simulink model "CM745A_Sci30CfgAndUse"  (R2013b)
settings: Solver=ode45  StartTime=0.0  StopTime=10.0  RelTol=1e-3
libraries: simulink x12
(part 2 of 3)

== system CM745A_Sci30CfgAndUse/Sci30CfgAndUse/Sci30CfgAndUsePer1/Update DTS registers/If Action Subsystem3 ==
  Action Port : ActionPort  ActionType=then
  Add1 : Sum  OutDataTypeStr=Inherit: Inherit via back propagation
  Constant : Constant  Value=0
  Constant1 : Constant  Value=0
  Constant4 : Constant  OutDataTypeStr=uint8
  CopyRight2 : Subsystem  Description=|  mask(Copyright Information){none=on}
      | Copyright info block.                                               
      |                                                                     
      | Place copyright information at the top of every subsystem in design.
      mask prompts: none "No parameters"
      mask help: Place copyright information at the top of every subsystem in design.
      mask Display:
      | NxtrConf = 'Nexteer Confidential';
      | 
      | sys = bdroot; %handle for the current model ("system")
      | first = get_param(sys,'Created');
      | first = first(end-3:end);  %year is last four digits
      | 
      | last = get_param(sys,'LastModifiedDate');
      | if isempty(last)
      |     last = datestr(now,'yyyy');
      | else
      |     last = last(end-3:end);
      | end
      | 
      | if strcmp(first,last)
      |     fprintf('%s -- Copyright %s Nexteer',NxtrConf,first)
      | else
      |     fprintf('%s -- %s%s- %s Nexteer',NxtrConf,char(169),first,last)
      | end
  Data Store Read5 : DataStoreRead  DataStoreName=SciDiagcOvrrunErrCntr
  Data Store Write3 : DataStoreWrite  DataStoreName=SciDiagcOvrrunErrCntr
  RegOutpSCI30ORER : Terminator
  RegOutpSCI30RDRF : Terminator
  wires:
  Constant/1 -> RegOutpSCI30ORER/1
  Constant1/1 -> RegOutpSCI30RDRF/1
  Data Store Read5/1 -> Add1/1
  Add1/1 -> Data Store Write3/1
  Constant4/1 -> Add1/2

== system CM745A_Sci30CfgAndUse/Sci30CfgAndUse/Sci30CfgAndUsePer1/Update DTS registers/If Action Subsystem4 ==
  Action Port : ActionPort  ActionType=then
  Add1 : Sum  OutDataTypeStr=Inherit: Inherit via back propagation
  Constant : Constant  Value=0
  Constant4 : Constant  OutDataTypeStr=uint8
  CopyRight2 : Subsystem  Description=|  mask(Copyright Information){none=on}
      | Copyright info block.                                               
      |                                                                     
      | Place copyright information at the top of every subsystem in design.
      mask prompts: none "No parameters"
      mask help: Place copyright information at the top of every subsystem in design.
      mask Display:
      | NxtrConf = 'Nexteer Confidential';
      | 
      | sys = bdroot; %handle for the current model ("system")
      | first = get_param(sys,'Created');
      | first = first(end-3:end);  %year is last four digits
      | 
      | last = get_param(sys,'LastModifiedDate');
      | if isempty(last)
      |     last = datestr(now,'yyyy');
      | else
      |     last = last(end-3:end);
      | end
      | 
      | if strcmp(first,last)
      |     fprintf('%s -- Copyright %s Nexteer',NxtrConf,first)
      | else
      |     fprintf('%s -- %s%s- %s Nexteer',NxtrConf,char(169),first,last)
      | end
  Data Store Read5 : DataStoreRead  DataStoreName=SciDiagcParErrCntr
  Data Store Write3 : DataStoreWrite  DataStoreName=SciDiagcParErrCntr
  RegOutpSCI30PER : Terminator
  wires:
  Constant/1 -> RegOutpSCI30PER/1
  Data Store Read5/1 -> Add1/1
  Add1/1 -> Data Store Write3/1
  Constant4/1 -> Add1/2

== system CM745A_Sci30CfgAndUse/Sci30CfgAndUse/Sci30CfgAndUsePer1/Update DTS registers/If Action Subsystem5 ==
  Action Port : ActionPort  ActionType=then
  Add1 : Sum  OutDataTypeStr=Inherit: Inherit via back propagation
  Constant : Constant  Value=0
  Constant4 : Constant  OutDataTypeStr=uint8
  CopyRight2 : Subsystem  Description=|  mask(Copyright Information){none=on}
      | Copyright info block.                                               
      |                                                                     
      | Place copyright information at the top of every subsystem in design.
      mask prompts: none "No parameters"
      mask help: Place copyright information at the top of every subsystem in design.
      mask Display:
      | NxtrConf = 'Nexteer Confidential';
      | 
      | sys = bdroot; %handle for the current model ("system")
      | first = get_param(sys,'Created');
      | first = first(end-3:end);  %year is last four digits
      | 
      | last = get_param(sys,'LastModifiedDate');
      | if isempty(last)
      |     last = datestr(now,'yyyy');
      | else
      |     last = last(end-3:end);
      | end
      | 
      | if strcmp(first,last)
      |     fprintf('%s -- Copyright %s Nexteer',NxtrConf,first)
      | else
      |     fprintf('%s -- %s%s- %s Nexteer',NxtrConf,char(169),first,last)
      | end
  Data Store Read5 : DataStoreRead  DataStoreName=SciDiagcFrmErrCntr
  Data Store Write3 : DataStoreWrite  DataStoreName=SciDiagcFrmErrCntr
  RegOutpSCI30FER : Terminator
  wires:
  Constant/1 -> RegOutpSCI30FER/1
  Data Store Read5/1 -> Add1/1
  Add1/1 -> Data Store Write3/1
  Constant4/1 -> Add1/2

== system CM745A_Sci30CfgAndUse/Sci30CfgAndUse/Sci30CfgAndUsePer2/GetTxRateGroup/CopyRight2 ==

== system CM745A_Sci30CfgAndUse/Sci30CfgAndUse/Sci30CfgAndUsePer2/Sci30Transmit/CopyRight2 ==

== system CM745A_Sci30CfgAndUse/Sci30CfgAndUse/Sci30CfgAndUsePer2/Sci30Transmit/If Action Subsystem ==
  Action Port : ActionPort  ActionType=then
  Constant : Constant  Value=0  OutDataTypeStr=boolean
  Constant1 : Constant  Value=0  OutDataTypeStr=uint8
  CopyRight2 : Subsystem  Description=|  mask(Copyright Information){none=on}
      | Copyright info block.                                               
      |                                                                     
      | Place copyright information at the top of every subsystem in design.
      mask prompts: none "No parameters"
      mask help: Place copyright information at the top of every subsystem in design.
      mask Display:
      | NxtrConf = 'Nexteer Confidential';
      | 
      | sys = bdroot; %handle for the current model ("system")
      | first = get_param(sys,'Created');
      | first = first(end-3:end);  %year is last four digits
      | 
      | last = get_param(sys,'LastModifiedDate');
      | if isempty(last)
      |     last = datestr(now,'yyyy');
      | else
      |     last = last(end-3:end);
      | end
      | 
      | if strcmp(first,last)
      |     fprintf('%s -- Copyright %s Nexteer',NxtrConf,first)
      | else
      |     fprintf('%s -- %s%s- %s Nexteer',NxtrConf,char(169),first,last)
      | end
  Data Store Write : DataStoreWrite  DataStoreName=SciTxSigGroupCnt
  Data Store Write1 : DataStoreWrite  DataStoreName=SciGlbTxCnt
  IMCARBN_NROF2MILLISECRATEGROUP_CNT_U08 : Constant  Value=0  OutDataTypeStr=uint8
  While Iterator Subsystem : Subsystem  TreatAsAtomicUnit=on
  wires:
  Constant/1 -> While Iterator Subsystem/1(IC)
  Constant1/1 -> Data Store Write/1
  IMCARBN_NROF2MILLISECRATEGROUP_CNT_U08/1 -> Data Store Write1/1

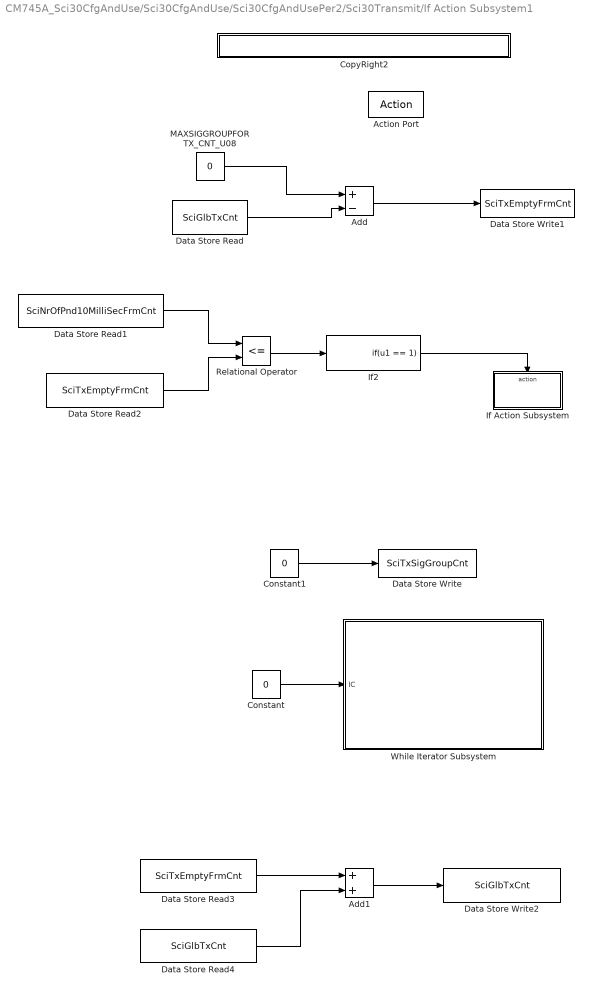
== system CM745A_Sci30CfgAndUse/Sci30CfgAndUse/Sci30CfgAndUsePer2/Sci30Transmit/If Action Subsystem1 ==
  Action Port : ActionPort  ActionType=then
  Add : Sum  Inputs=+-
  Add1 : Sum
  Constant : Constant  Value=0  OutDataTypeStr=boolean
  Constant1 : Constant  Value=0  OutDataTypeStr=uint8
  CopyRight2 : Subsystem  Description=|  mask(Copyright Information){none=on}
      | Copyright info block.                                               
      |                                                                     
      | Place copyright information at the top of every subsystem in design.
      mask prompts: none "No parameters"
      mask help: Place copyright information at the top of every subsystem in design.
      mask Display:
      | NxtrConf = 'Nexteer Confidential';
      | 
      | sys = bdroot; %handle for the current model ("system")
      | first = get_param(sys,'Created');
      | first = first(end-3:end);  %year is last four digits
      | 
      | last = get_param(sys,'LastModifiedDate');
      | if isempty(last)
      |     last = datestr(now,'yyyy');
      | else
      |     last = last(end-3:end);
      | end
      | 
      | if strcmp(first,last)
      |     fprintf('%s -- Copyright %s Nexteer',NxtrConf,first)
      | else
      |     fprintf('%s -- %s%s- %s Nexteer',NxtrConf,char(169),first,last)
      | end
  Data Store Read : DataStoreRead  DataStoreName=SciGlbTxCnt
  Data Store Read1 : DataStoreRead  DataStoreName=SciNrOfPnd10MilliSecFrmCnt
  Data Store Read2 : DataStoreRead  DataStoreName=SciTxEmptyFrmCnt
  Data Store Read3 : DataStoreRead  DataStoreName=SciTxEmptyFrmCnt
  Data Store Read4 : DataStoreRead  DataStoreName=SciGlbTxCnt
  Data Store Write : DataStoreWrite  DataStoreName=SciTxSigGroupCnt
  Data Store Write1 : DataStoreWrite  DataStoreName=SciTxEmptyFrmCnt
  Data Store Write2 : DataStoreWrite  DataStoreName=SciGlbTxCnt
  If Action Subsystem : Subsystem  TreatAsAtomicUnit=on
  If2 : If  IfExpression=u1 == 1  ShowElse=off
      settings: AttributesFormatString=%<IfExpression>
  MAXSIGGROUPFORTX_CNT_U08 : Constant  Value=0  OutDataTypeStr=uint8
  Relational Operator : RelationalOperator  Operator=<=  OutDataTypeStr=boolean
  While Iterator Subsystem : Subsystem  TreatAsAtomicUnit=on
  wires:
  Constant/1 -> While Iterator Subsystem/1(IC)
  Constant1/1 -> Data Store Write/1
  MAXSIGGROUPFORTX_CNT_U08/1 -> Add/1
  Data Store Read/1 -> Add/2
  Add/1 -> Data Store Write1/1
  Relational Operator/1 -> If2/1
  Data Store Read1/1 -> Relational Operator/1
  Data Store Read2/1 -> Relational Operator/2
  If2/1 -> If Action Subsystem/Action
  Data Store Read4/1 -> Add1/2
  Data Store Read3/1 -> Add1/1
  Add1/1 -> Data Store Write2/1

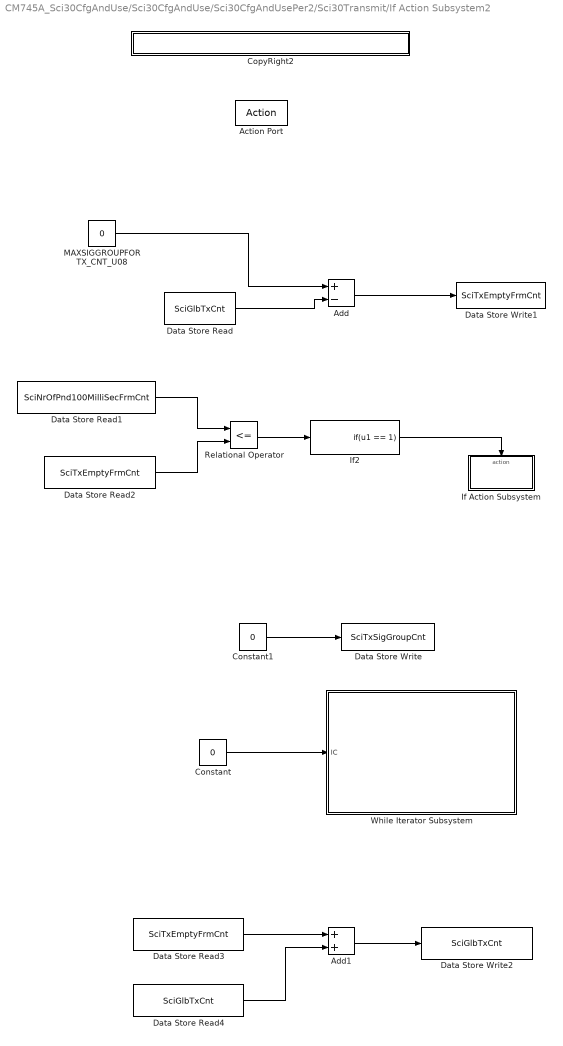
== system CM745A_Sci30CfgAndUse/Sci30CfgAndUse/Sci30CfgAndUsePer2/Sci30Transmit/If Action Subsystem2 ==
  Action Port : ActionPort  ActionType=then
  Add : Sum  Inputs=+-
  Add1 : Sum
  Constant : Constant  Value=0  OutDataTypeStr=boolean
  Constant1 : Constant  Value=0  OutDataTypeStr=uint8
  CopyRight2 : Subsystem  Description=|  mask(Copyright Information){none=on}
      | Copyright info block.                                               
      |                                                                     
      | Place copyright information at the top of every subsystem in design.
      mask prompts: none "No parameters"
      mask help: Place copyright information at the top of every subsystem in design.
      mask Display:
      | NxtrConf = 'Nexteer Confidential';
      | 
      | sys = bdroot; %handle for the current model ("system")
      | first = get_param(sys,'Created');
      | first = first(end-3:end);  %year is last four digits
      | 
      | last = get_param(sys,'LastModifiedDate');
      | if isempty(last)
      |     last = datestr(now,'yyyy');
      | else
      |     last = last(end-3:end);
      | end
      | 
      | if strcmp(first,last)
      |     fprintf('%s -- Copyright %s Nexteer',NxtrConf,first)
      | else
      |     fprintf('%s -- %s%s- %s Nexteer',NxtrConf,char(169),first,last)
      | end
  Data Store Read : DataStoreRead  DataStoreName=SciGlbTxCnt
  Data Store Read1 : DataStoreRead  DataStoreName=SciNrOfPnd100MilliSecFrmCnt
  Data Store Read2 : DataStoreRead  DataStoreName=SciTxEmptyFrmCnt
  Data Store Read3 : DataStoreRead  DataStoreName=SciTxEmptyFrmCnt
  Data Store Read4 : DataStoreRead  DataStoreName=SciGlbTxCnt
  Data Store Write : DataStoreWrite  DataStoreName=SciTxSigGroupCnt
  Data Store Write1 : DataStoreWrite  DataStoreName=SciTxEmptyFrmCnt
  Data Store Write2 : DataStoreWrite  DataStoreName=SciGlbTxCnt
  If Action Subsystem : Subsystem  TreatAsAtomicUnit=on
  If2 : If  IfExpression=u1 == 1  ShowElse=off
      settings: AttributesFormatString=%<IfExpression>
  MAXSIGGROUPFORTX_CNT_U08 : Constant  Value=0  VectorParams1D=off  OutDataTypeStr=uint8
  Relational Operator : RelationalOperator  Operator=<=  OutDataTypeStr=boolean
  While Iterator Subsystem : Subsystem  TreatAsAtomicUnit=on
  wires:
  Constant/1 -> While Iterator Subsystem/1(IC)
  Constant1/1 -> Data Store Write/1
  Data Store Read/1 -> Add/2
  Add/1 -> Data Store Write1/1
  Relational Operator/1 -> If2/1
  Data Store Read1/1 -> Relational Operator/1
  Data Store Read2/1 -> Relational Operator/2
  If2/1 -> If Action Subsystem/Action
  Data Store Read4/1 -> Add1/2
  Data Store Read3/1 -> Add1/1
  Add1/1 -> Data Store Write2/1
  MAXSIGGROUPFORTX_CNT_U08/1 -> Add/1

== system CM745A_Sci30CfgAndUse/Sci30CfgAndUse/Sci30CfgAndUsePer2/Sci30Transmit/Update DTS registers ==
  note: Following register writes correspond to SCI30TX
  Constant5 : Constant  Value=0  OutDataTypeStr=uint8
  Constant6 : Constant  OutDataTypeStr=uint8
  CopyRight2 : Subsystem  Description=|  mask(Copyright Information){none=on}
      | Copyright info block.                                               
      |                                                                     
      | Place copyright information at the top of every subsystem in design.
      mask prompts: none "No parameters"
      mask help: Place copyright information at the top of every subsystem in design.
      mask Display:
      | NxtrConf = 'Nexteer Confidential';
      | 
      | sys = bdroot; %handle for the current model ("system")
      | first = get_param(sys,'Created');
      | first = first(end-3:end);  %year is last four digits
      | 
      | last = get_param(sys,'LastModifiedDate');
      | if isempty(last)
      |     last = datestr(now,'yyyy');
      | else
      |     last = last(end-3:end);
      | end
      | 
      | if strcmp(first,last)
      |     fprintf('%s -- Copyright %s Nexteer',NxtrConf,first)
      | else
      |     fprintf('%s -- %s%s- %s Nexteer',NxtrConf,char(169),first,last)
      | end
  Data Store Read4 : DataStoreRead  DataStoreName=SciGlbTxCnt
  If : If  NumInputs=2  IfExpression=u1 == 1 & u2 == 1  ShowElse=off
  If Action Subsystem : Subsystem  TreatAsAtomicUnit=on
  RegInpSCI30TDRE : Ground
  Relational Operator : RelationalOperator  Operator=>  OutDataTypeStr=boolean
  Relational Operator1 : RelationalOperator  Operator===  OutDataTypeStr=boolean
  wires:
  Data Store Read4/1 -> Relational Operator/1
  Constant5/1 -> Relational Operator/2
  Relational Operator/1 -> If/1
  If/1 -> If Action Subsystem/Action
  RegInpSCI30TDRE/1 -> Relational Operator1/1
  Constant6/1 -> Relational Operator1/2
  Relational Operator1/1 -> If/2

== system CM745A_Sci30CfgAndUse/Sci30CfgAndUse/Sci30CfgAndUsePer3/GetTxRateGroup/CopyRight2 ==

== system CM745A_Sci30CfgAndUse/Sci30CfgAndUse/Sci30CfgAndUsePer4/GetTxRateGroup/CopyRight2 ==

== system CM745A_Sci30CfgAndUse/Sci30CfgAndUse/Sci30CfgAndUsePer1/If Action Subsystem2/While Iterator Subsystem/CopyRight2 ==

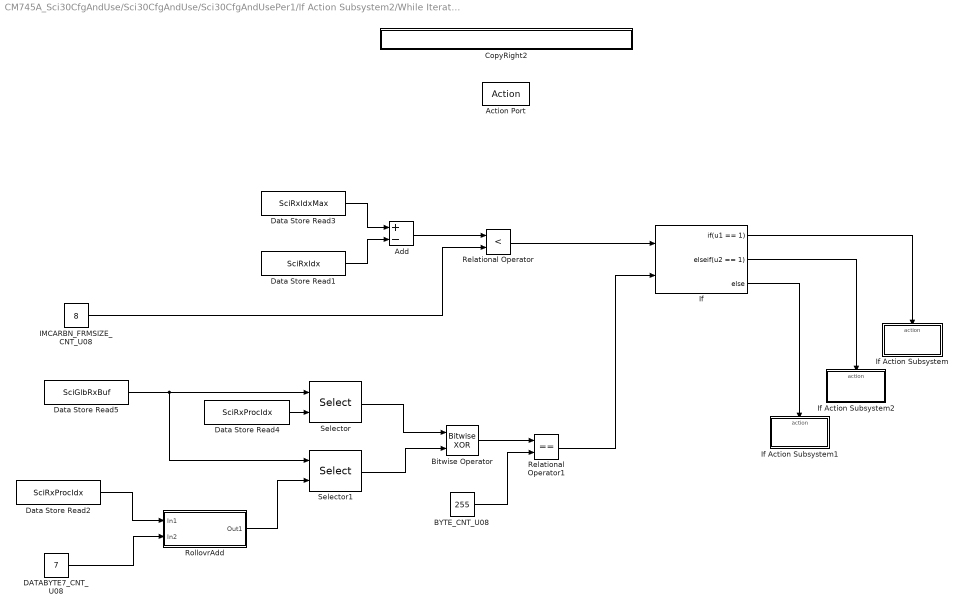
== system CM745A_Sci30CfgAndUse/Sci30CfgAndUse/Sci30CfgAndUsePer1/If Action Subsystem2/While Iterator Subsystem/If Action Subsystem ==
  Action Port : ActionPort  ActionType=then
  Add : Sum  Inputs=+-
  BYTE_CNT_U08 : Constant  Value=255  OutDataTypeStr=uint8
  Bitwise Operator : simulink/Logic and Bit Operations/Bitwise Operator  logicop=XOR  UseBitMask=off  NumInputPorts=2  BitMask=bin2dec('11011001')  BitMaskRealWorld=Stored Integer
  CopyRight2 : Subsystem  Description=|  mask(Copyright Information){none=on}
      | Copyright info block.                                               
      |                                                                     
      | Place copyright information at the top of every subsystem in design.
      mask prompts: none "No parameters"
      mask help: Place copyright information at the top of every subsystem in design.
      mask Display:
      | NxtrConf = 'Nexteer Confidential';
      | 
      | sys = bdroot; %handle for the current model ("system")
      | first = get_param(sys,'Created');
      | first = first(end-3:end);  %year is last four digits
      | 
      | last = get_param(sys,'LastModifiedDate');
      | if isempty(last)
      |     last = datestr(now,'yyyy');
      | else
      |     last = last(end-3:end);
      | end
      | 
      | if strcmp(first,last)
      |     fprintf('%s -- Copyright %s Nexteer',NxtrConf,first)
      | else
      |     fprintf('%s -- %s%s- %s Nexteer',NxtrConf,char(169),first,last)
      | end
  DATABYTE7_CNT_U08 : Constant  Value=7
  Data Store Read1 : DataStoreRead  DataStoreName=SciRxIdx
  Data Store Read2 : DataStoreRead  DataStoreName=SciRxProcIdx
  Data Store Read3 : DataStoreRead  DataStoreName=SciRxIdxMax
  Data Store Read4 : DataStoreRead  DataStoreName=SciRxProcIdx
  Data Store Read5 : DataStoreRead  DataStoreName=SciGlbRxBuf
  IMCARBN_FRMSIZE_CNT_U08 : Constant  Value=8
  If : If  NumInputs=2  IfExpression=u1 == 1  ElseIfExpressions=u2 == 1
      settings: AttributesFormatString=|
      | %<ElseIfExpressions>
      | %<IfExpression>
  If Action Subsystem : Subsystem  TreatAsAtomicUnit=on
  If Action Subsystem1 : Subsystem  TreatAsAtomicUnit=on
  If Action Subsystem2 : Subsystem  TreatAsAtomicUnit=on
  Relational Operator : RelationalOperator  Operator=<  OutDataTypeStr=boolean
  Relational Operator1 : RelationalOperator  Operator===  OutDataTypeStr=boolean
  RollovrAdd : Subsystem
  Selector : Selector  IndexMode=Zero-based  InputPortWidth=8  IndexOptions=Index vector (port)  Indices=[0]  OutputSizes=1
  Selector1 : Selector  IndexMode=Zero-based  InputPortWidth=8  IndexOptions=Index vector (port)  Indices=[0]  OutputSizes=1
  wires:
  If/1 -> If Action Subsystem/Action
  Relational Operator1/1 -> If/2
  Relational Operator/1 -> If/1
  Data Store Read3/1 -> Add/1
  Data Store Read1/1 -> Add/2
  Add/1 -> Relational Operator/1
  RollovrAdd/1(Out1) -> Selector1/2
  Data Store Read2/1 -> RollovrAdd/1(In1)
  IMCARBN_FRMSIZE_CNT_U08/1 -> Relational Operator/2
  Selector1/1 -> Bitwise Operator/2
  Data Store Read5/1 -> Selector1/1, Selector/1
  Selector/1 -> Bitwise Operator/1
  Data Store Read4/1 -> Selector/2
  BYTE_CNT_U08/1 -> Relational Operator1/2
  Bitwise Operator/1 -> Relational Operator1/1
  If/2 -> If Action Subsystem2/Action
  If/3 -> If Action Subsystem1/Action
  DATABYTE7_CNT_U08/1 -> RollovrAdd/2(In2)

== system CM745A_Sci30CfgAndUse/Sci30CfgAndUse/Sci30CfgAndUsePer1/If Action Subsystem2/While Iterator Subsystem/If Action Subsystem1 ==
  Action Port : ActionPort  ActionType=else
  Constant : Constant  OutDataTypeStr=uint8
  CopyRight2 : Subsystem  Description=|  mask(Copyright Information){none=on}
      | Copyright info block.                                               
      |                                                                     
      | Place copyright information at the top of every subsystem in design.
      mask prompts: none "No parameters"
      mask help: Place copyright information at the top of every subsystem in design.
      mask Display:
      | NxtrConf = 'Nexteer Confidential';
      | 
      | sys = bdroot; %handle for the current model ("system")
      | first = get_param(sys,'Created');
      | first = first(end-3:end);  %year is last four digits
      | 
      | last = get_param(sys,'LastModifiedDate');
      | if isempty(last)
      |     last = datestr(now,'yyyy');
      | else
      |     last = last(end-3:end);
      | end
      | 
      | if strcmp(first,last)
      |     fprintf('%s -- Copyright %s Nexteer',NxtrConf,first)
      | else
      |     fprintf('%s -- %s%s- %s Nexteer',NxtrConf,char(169),first,last)
      | end
  Data Store Read2 : DataStoreRead  DataStoreName=SciRxProcIdx
  Data Store Write : DataStoreWrite  DataStoreName=SciRxProcIdx
  RollovrAdd : Subsystem
  wires:
  RollovrAdd/1(Out1) -> Data Store Write/1
  Data Store Read2/1 -> RollovrAdd/1(In1)
  Constant/1 -> RollovrAdd/2(In2)

== system CM745A_Sci30CfgAndUse/Sci30CfgAndUse/Sci30CfgAndUsePer1/If Action Subsystem2/While Iterator Subsystem/RollovrAdd ==
  In1 : Inport
  In2 : Inport  Port=2
  Add : Sum
  Constant : Constant  Value=2  OutDataTypeStr=uint8
  CopyRight2 : Subsystem  Description=|  mask(Copyright Information){none=on}
      | Copyright info block.                                               
      |                                                                     
      | Place copyright information at the top of every subsystem in design.
      mask prompts: none "No parameters"
      mask help: Place copyright information at the top of every subsystem in design.
      mask Display:
      | NxtrConf = 'Nexteer Confidential';
      | 
      | sys = bdroot; %handle for the current model ("system")
      | first = get_param(sys,'Created');
      | first = first(end-3:end);  %year is last four digits
      | 
      | last = get_param(sys,'LastModifiedDate');
      | if isempty(last)
      |     last = datestr(now,'yyyy');
      | else
      |     last = last(end-3:end);
      | end
      | 
      | if strcmp(first,last)
      |     fprintf('%s -- Copyright %s Nexteer',NxtrConf,first)
      | else
      |     fprintf('%s -- %s%s- %s Nexteer',NxtrConf,char(169),first,last)
      | end
  IMCARBN_FRMSIZE_CNT_U08 : Constant  Value=8  OutDataTypeStr=uint8
  MAXSIGGROUPFORTX_CNT_U08 : Constant  Value=9  OutDataTypeStr=uint8
  Math Function : Math  Operator=mod  SaturateOnIntegerOverflow=on
  Product : Product
  Product1 : Product  OutDataTypeStr=uint8
  Out1 : Outport
  wires:
  Math Function/1 -> Out1/1
  In1/1 -> Add/1
  In2/1 -> Add/2
  Add/1 -> Math Function/1
  Constant/1 -> Product/1
  IMCARBN_FRMSIZE_CNT_U08/1 -> Product/2
  Product/1 -> Product1/1
  Product1/1 -> Math Function/2
  MAXSIGGROUPFORTX_CNT_U08/1 -> Product1/2

== system CM745A_Sci30CfgAndUse/Sci30CfgAndUse/Sci30CfgAndUsePer1/Update DTS registers/If Action Subsystem1/CopyRight2 ==

== system CM745A_Sci30CfgAndUse/Sci30CfgAndUse/Sci30CfgAndUsePer1/Update DTS registers/If Action Subsystem3/CopyRight2 ==

== system CM745A_Sci30CfgAndUse/Sci30CfgAndUse/Sci30CfgAndUsePer1/Update DTS registers/If Action Subsystem4/CopyRight2 ==

== system CM745A_Sci30CfgAndUse/Sci30CfgAndUse/Sci30CfgAndUsePer1/Update DTS registers/If Action Subsystem5/CopyRight2 ==

== system CM745A_Sci30CfgAndUse/Sci30CfgAndUse/Sci30CfgAndUsePer2/Sci30Transmit/If Action Subsystem/CopyRight2 ==

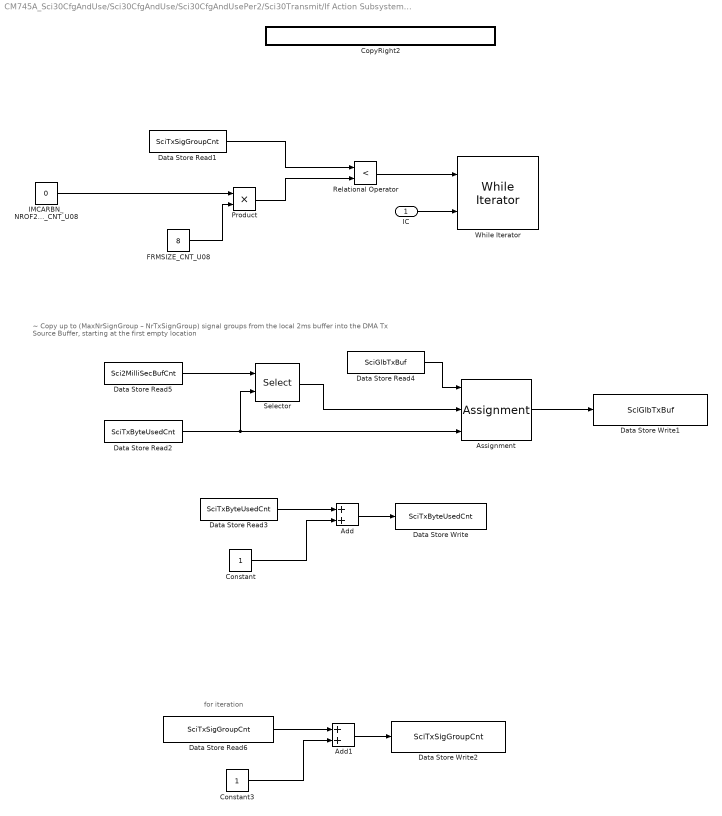
== system CM745A_Sci30CfgAndUse/Sci30CfgAndUse/Sci30CfgAndUsePer2/Sci30Transmit/If Action Subsystem/While Iterator Subsystem ==
  note: ~ Copy up to (MaxNrSignGroup – NrTxSignGroup) signal groups from the local 2ms buffer into the DMA Tx Source Buffer, starting at the first empty location
  note: for iteration
  IC : Inport
  Add : Sum
  Add1 : Sum
  Assignment : Assignment  IndexMode=Zero-based  IndexOptions=Index vector (port)  Indices=1  OutputSizes=1
  Constant : Constant  OutDataTypeStr=uint8
  Constant3 : Constant  OutDataTypeStr=uint8
  CopyRight2 : Subsystem  Description=|  mask(Copyright Information){none=on}
      | Copyright info block.                                               
      |                                                                     
      | Place copyright information at the top of every subsystem in design.
      mask prompts: none "No parameters"
      mask help: Place copyright information at the top of every subsystem in design.
      mask Display:
      | NxtrConf = 'Nexteer Confidential';
      | 
      | sys = bdroot; %handle for the current model ("system")
      | first = get_param(sys,'Created');
      | first = first(end-3:end);  %year is last four digits
      | 
      | last = get_param(sys,'LastModifiedDate');
      | if isempty(last)
      |     last = datestr(now,'yyyy');
      | else
      |     last = last(end-3:end);
      | end
      | 
      | if strcmp(first,last)
      |     fprintf('%s -- Copyright %s Nexteer',NxtrConf,first)
      | else
      |     fprintf('%s -- %s%s- %s Nexteer',NxtrConf,char(169),first,last)
      | end
  Data Store Read1 : DataStoreRead  DataStoreName=SciTxSigGroupCnt
  Data Store Read2 : DataStoreRead  DataStoreName=SciTxByteUsedCnt
  Data Store Read3 : DataStoreRead  DataStoreName=SciTxByteUsedCnt
  Data Store Read4 : DataStoreRead  DataStoreName=SciGlbTxBuf
  Data Store Read5 : DataStoreRead  DataStoreName=Sci2MilliSecBufCnt
  Data Store Read6 : DataStoreRead  DataStoreName=SciTxSigGroupCnt
  Data Store Write : DataStoreWrite  DataStoreName=SciTxByteUsedCnt
  Data Store Write1 : DataStoreWrite  DataStoreName=SciGlbTxBuf
  Data Store Write2 : DataStoreWrite  DataStoreName=SciTxSigGroupCnt
  FRMSIZE_CNT_U08 : Constant  Value=8  OutDataTypeStr=uint8
  IMCARBN_NROF2MILLISECRATEGROUP_CNT_U08 : Constant  Value=0
  Product : Product
  Relational Operator : RelationalOperator  Operator=<  OutDataTypeStr=boolean
  Selector : Selector  IndexMode=Zero-based  InputPortWidth=2047  IndexOptions=Index vector (port)  Indices=[1 3]  OutputSizes=1
  While Iterator : WhileIterator  MaxIters=-1  ResetStates=reset
  wires:
  IC/1 -> While Iterator/2
  Data Store Read1/1 -> Relational Operator/1
  IMCARBN_NROF2MILLISECRATEGROUP_CNT_U08/1 -> Product/1
  FRMSIZE_CNT_U08/1 -> Product/2
  Product/1 -> Relational Operator/2
  Relational Operator/1 -> While Iterator/1
  Data Store Read3/1 -> Add/1
  Add/1 -> Data Store Write/1
  Constant/1 -> Add/2
  Assignment/1 -> Data Store Write1/1
  Data Store Read2/1 -> Selector/2, Assignment/3
  Data Store Read4/1 -> Assignment/1
  Selector/1 -> Assignment/2
  Data Store Read5/1 -> Selector/1
  Data Store Read6/1 -> Add1/1
  Add1/1 -> Data Store Write2/1
  Constant3/1 -> Add1/2

== system CM745A_Sci30CfgAndUse/Sci30CfgAndUse/Sci30CfgAndUsePer2/Sci30Transmit/If Action Subsystem1/CopyRight2 ==

== system CM745A_Sci30CfgAndUse/Sci30CfgAndUse/Sci30CfgAndUsePer2/Sci30Transmit/If Action Subsystem1/If Action Subsystem ==
  Action Port : ActionPort  ActionType=then
  Constant : Constant  Value=0  OutDataTypeStr=boolean
  CopyRight2 : Subsystem  Description=|  mask(Copyright Information){none=on}
      | Copyright info block.                                               
      |                                                                     
      | Place copyright information at the top of every subsystem in design.
      mask prompts: none "No parameters"
      mask help: Place copyright information at the top of every subsystem in design.
      mask Display:
      | NxtrConf = 'Nexteer Confidential';
      | 
      | sys = bdroot; %handle for the current model ("system")
      | first = get_param(sys,'Created');
      | first = first(end-3:end);  %year is last four digits
      | 
      | last = get_param(sys,'LastModifiedDate');
      | if isempty(last)
      |     last = datestr(now,'yyyy');
      | else
      |     last = last(end-3:end);
      | end
      | 
      | if strcmp(first,last)
      |     fprintf('%s -- Copyright %s Nexteer',NxtrConf,first)
      | else
      |     fprintf('%s -- %s%s- %s Nexteer',NxtrConf,char(169),first,last)
      | end
  Data Store Read1 : DataStoreRead  DataStoreName=SciNrOfPnd10MilliSecFrmCnt
  Data Store Write1 : DataStoreWrite  DataStoreName=SciTxEmptyFrmCnt
  Data Store Write2 : DataStoreWrite  DataStoreName=Sci10MilliSecReadCmpl
  wires:
  Data Store Read1/1 -> Data Store Write1/1
  Constant/1 -> Data Store Write2/1

== system CM745A_Sci30CfgAndUse/Sci30CfgAndUse/Sci30CfgAndUsePer2/Sci30Transmit/If Action Subsystem1/While Iterator Subsystem ==
  note: for iteration
  IC : Inport
  Add : Sum  Inputs=+-
  Add1 : Sum
  Constant : Constant  OutDataTypeStr=uint8
  Constant1 : Constant  Value=0  OutDataTypeStr=boolean
  Constant2 : Constant  Value=0  OutDataTypeStr=uint8
  Constant3 : Constant  OutDataTypeStr=uint8
  CopyRight2 : Subsystem  Description=|  mask(Copyright Information){none=on}
      | Copyright info block.                                               
      |                                                                     
      | Place copyright information at the top of every subsystem in design.
      mask prompts: none "No parameters"
      mask help: Place copyright information at the top of every subsystem in design.
      mask Display:
      | NxtrConf = 'Nexteer Confidential';
      | 
      | sys = bdroot; %handle for the current model ("system")
      | first = get_param(sys,'Created');
      | first = first(end-3:end);  %year is last four digits
      | 
      | last = get_param(sys,'LastModifiedDate');
      | if isempty(last)
      |     last = datestr(now,'yyyy');
      | else
      |     last = last(end-3:end);
      | end
      | 
      | if strcmp(first,last)
      |     fprintf('%s -- Copyright %s Nexteer',NxtrConf,first)
      | else
      |     fprintf('%s -- %s%s- %s Nexteer',NxtrConf,char(169),first,last)
      | end
  Data Store Read1 : DataStoreRead  DataStoreName=SciTxSigGroupCnt
  Data Store Read2 : DataStoreRead  DataStoreName=SciTxSigGroupCnt
  Data Store Read3 : DataStoreRead  DataStoreName=SciNrOfPnd10MilliSecFrmCnt
  Data Store Read6 : DataStoreRead  DataStoreName=SciTxEmptyFrmCnt
  Data Store Write : DataStoreWrite  DataStoreName=SciNrOfPnd10MilliSecFrmCnt
  Data Store Write1 : DataStoreWrite  DataStoreName=SciTxSigByteCnt
  Data Store Write2 : DataStoreWrite  DataStoreName=SciTxSigGroupCnt
  Relational Operator : RelationalOperator  Operator=<  OutDataTypeStr=boolean
  While Iterator : WhileIterator  MaxIters=-1  ResetStates=reset
  While Iterator Subsystem : Subsystem  TreatAsAtomicUnit=on
  wires:
  IC/1 -> While Iterator/2
  Data Store Read1/1 -> Relational Operator/1
  Relational Operator/1 -> While Iterator/1
  Data Store Read3/1 -> Add/1
  Add/1 -> Data Store Write/1
  Constant/1 -> Add/2
  Data Store Read6/1 -> Relational Operator/2
  Constant1/1 -> While Iterator Subsystem/1(IC)
  Constant2/1 -> Data Store Write1/1
  Data Store Read2/1 -> Add1/1
  Add1/1 -> Data Store Write2/1
  Constant3/1 -> Add1/2

== system CM745A_Sci30CfgAndUse/Sci30CfgAndUse/Sci30CfgAndUsePer2/Sci30Transmit/If Action Subsystem2/CopyRight2 ==

== system CM745A_Sci30CfgAndUse/Sci30CfgAndUse/Sci30CfgAndUsePer2/Sci30Transmit/If Action Subsystem2/If Action Subsystem ==
  Action Port : ActionPort  ActionType=then
  Constant : Constant  Value=0  OutDataTypeStr=boolean
  CopyRight2 : Subsystem  Description=|  mask(Copyright Information){none=on}
      | Copyright info block.                                               
      |                                                                     
      | Place copyright information at the top of every subsystem in design.
      mask prompts: none "No parameters"
      mask help: Place copyright information at the top of every subsystem in design.
      mask Display:
      | NxtrConf = 'Nexteer Confidential';
      | 
      | sys = bdroot; %handle for the current model ("system")
      | first = get_param(sys,'Created');
      | first = first(end-3:end);  %year is last four digits
      | 
      | last = get_param(sys,'LastModifiedDate');
      | if isempty(last)
      |     last = datestr(now,'yyyy');
      | else
      |     last = last(end-3:end);
      | end
      | 
      | if strcmp(first,last)
      |     fprintf('%s -- Copyright %s Nexteer',NxtrConf,first)
      | else
      |     fprintf('%s -- %s%s- %s Nexteer',NxtrConf,char(169),first,last)
      | end
  Data Store Read1 : DataStoreRead  DataStoreName=SciNrOfPnd100MilliSecFrmCnt
  Data Store Write1 : DataStoreWrite  DataStoreName=SciTxEmptyFrmCnt
  Data Store Write2 : DataStoreWrite  DataStoreName=Sci100MilliSecReadCmpl
  wires:
  Data Store Read1/1 -> Data Store Write1/1
  Constant/1 -> Data Store Write2/1

== system CM745A_Sci30CfgAndUse/Sci30CfgAndUse/Sci30CfgAndUsePer2/Sci30Transmit/If Action Subsystem2/While Iterator Subsystem ==
  note: for iteration
  IC : Inport
  Add : Sum  Inputs=+-
  Add1 : Sum
  Constant : Constant  OutDataTypeStr=uint8
  Constant1 : Constant  Value=0  OutDataTypeStr=boolean
  Constant2 : Constant  Value=0  OutDataTypeStr=uint8
  Constant3 : Constant  OutDataTypeStr=uint8
  CopyRight2 : Subsystem  Description=|  mask(Copyright Information){none=on}
      | Copyright info block.                                               
      |                                                                     
      | Place copyright information at the top of every subsystem in design.
      mask prompts: none "No parameters"
      mask help: Place copyright information at the top of every subsystem in design.
      mask Display:
      | NxtrConf = 'Nexteer Confidential';
      | 
      | sys = bdroot; %handle for the current model ("system")
      | first = get_param(sys,'Created');
      | first = first(end-3:end);  %year is last four digits
      | 
      | last = get_param(sys,'LastModifiedDate');
      | if isempty(last)
      |     last = datestr(now,'yyyy');
      | else
      |     last = last(end-3:end);
      | end
      | 
      | if strcmp(first,last)
      |     fprintf('%s -- Copyright %s Nexteer',NxtrConf,first)
      | else
      |     fprintf('%s -- %s%s- %s Nexteer',NxtrConf,char(169),first,last)
      | end
  Data Store Read1 : DataStoreRead  DataStoreName=SciTxSigGroupCnt
  Data Store Read2 : DataStoreRead  DataStoreName=SciTxSigGroupCnt
  Data Store Read3 : DataStoreRead  DataStoreName=SciNrOfPnd100MilliSecFrmCnt
  Data Store Read6 : DataStoreRead  DataStoreName=SciTxEmptyFrmCnt
  Data Store Write : DataStoreWrite  DataStoreName=SciNrOfPnd100MilliSecFrmCnt
  Data Store Write1 : DataStoreWrite  DataStoreName=SciTxSigByteCnt
  Data Store Write2 : DataStoreWrite  DataStoreName=SciTxSigGroupCnt
  Relational Operator : RelationalOperator  Operator=<  OutDataTypeStr=boolean
  While Iterator : WhileIterator  MaxIters=-1  ResetStates=reset
  While Iterator Subsystem : Subsystem  TreatAsAtomicUnit=on
  wires:
  IC/1 -> While Iterator/2
  Data Store Read1/1 -> Relational Operator/1
  Relational Operator/1 -> While Iterator/1
  Data Store Read3/1 -> Add/1
  Add/1 -> Data Store Write/1
  Constant/1 -> Add/2
  Data Store Read6/1 -> Relational Operator/2
  Constant1/1 -> While Iterator Subsystem/1(IC)
  Constant2/1 -> Data Store Write1/1
  Data Store Read2/1 -> Add1/1
  Add1/1 -> Data Store Write2/1
  Constant3/1 -> Add1/2

== system CM745A_Sci30CfgAndUse/Sci30CfgAndUse/Sci30CfgAndUsePer2/Sci30Transmit/Update DTS registers/CopyRight2 ==

== system CM745A_Sci30CfgAndUse/Sci30CfgAndUse/Sci30CfgAndUsePer2/Sci30Transmit/Update DTS registers/If Action Subsystem ==
  note: DMASSDTDA088 = (uint32)&SCI30TDR;
  note: DMASSDTSA088 = (uint32)&SciGlbTxBuf[0];
  Action Port : ActionPort  ActionType=then
  Constant : Constant  Value=0  OutDataTypeStr=uint8
  Constant1 : Constant
  Constant2 : Constant
  Constant3 : Constant  Value=0
  Constant4 : Constant
  CopyRight2 : Subsystem  Description=|  mask(Copyright Information){none=on}
      | Copyright info block.                                               
      |                                                                     
      | Place copyright information at the top of every subsystem in design.
      mask prompts: none "No parameters"
      mask help: Place copyright information at the top of every subsystem in design.
      mask Display:
      | NxtrConf = 'Nexteer Confidential';
      | 
      | sys = bdroot; %handle for the current model ("system")
      | first = get_param(sys,'Created');
      | first = first(end-3:end);  %year is last four digits
      | 
      | last = get_param(sys,'LastModifiedDate');
      | if isempty(last)
      |     last = datestr(now,'yyyy');
      | else
      |     last = last(end-3:end);
      | end
      | 
      | if strcmp(first,last)
      |     fprintf('%s -- Copyright %s Nexteer',NxtrConf,first)
      | else
      |     fprintf('%s -- %s%s- %s Nexteer',NxtrConf,char(169),first,last)
      | end
  Data Store Read3 : DataStoreRead  DataStoreName=SciGlbTxCnt
  Data Store Write1 : DataStoreWrite  DataStoreName=SciGlbTxCnt
  IMCARBN_FRMSIZE_CNT_U08 : Constant  Value=8  OutDataTypeStr=uint8
  Product : Product  OutDataTypeStr=uint8
  RegOutpDMASSDTFSC088 : Terminator
  RegOutpDMASSDTFSL088 : Terminator
  "RegOutpDMASSDTFSL088 " : Terminator
  RegOutpDMASSDTFSS088 : Terminator
  RegOutpDMASSDTTC088 : Terminator
  wires:
  Data Store Read3/1 -> Product/1
  IMCARBN_FRMSIZE_CNT_U08/1 -> Product/2
  Product/1 -> RegOutpDMASSDTTC088/1
  Constant/1 -> Data Store Write1/1
  Constant3/1 -> RegOutpDMASSDTFSL088/1
  Constant4/1 -> RegOutpDMASSDTFSC088/1
  Constant1/1 -> "RegOutpDMASSDTFSL088 "/1
  Constant2/1 -> RegOutpDMASSDTFSS088/1

== system CM745A_Sci30CfgAndUse/Sci30CfgAndUse/Sci30CfgAndUsePer1/If Action Subsystem2/While Iterator Subsystem/If Action Subsystem/CopyRight2 ==

== system CM745A_Sci30CfgAndUse/Sci30CfgAndUse/Sci30CfgAndUsePer1/If Action Subsystem2/While Iterator Subsystem/If Action Subsystem/If Action Subsystem ==
  Action Port : ActionPort  ActionType=then
  Add : Sum  Inputs=+-
  Constant : Constant  OutDataTypeStr=boolean
  CopyRight2 : Subsystem  Description=|  mask(Copyright Information){none=on}
      | Copyright info block.                                               
      |                                                                     
      | Place copyright information at the top of every subsystem in design.
      mask prompts: none "No parameters"
      mask help: Place copyright information at the top of every subsystem in design.
      mask Display:
      | NxtrConf = 'Nexteer Confidential';
      | 
      | sys = bdroot; %handle for the current model ("system")
      | first = get_param(sys,'Created');
      | first = first(end-3:end);  %year is last four digits
      | 
      | last = get_param(sys,'LastModifiedDate');
      | if isempty(last)
      |     last = datestr(now,'yyyy');
      | else
      |     last = last(end-3:end);
      | end
      | 
      | if strcmp(first,last)
      |     fprintf('%s -- Copyright %s Nexteer',NxtrConf,first)
      | else
      |     fprintf('%s -- %s%s- %s Nexteer',NxtrConf,char(169),first,last)
      | end
  Data Store Read1 : DataStoreRead  DataStoreName=SciRxIdx
  Data Store Read3 : DataStoreRead  DataStoreName=SciRxIdxMax
  Data Store Write : DataStoreWrite  DataStoreName=SciRxSetBreakLoop
  Data Store Write1 : DataStoreWrite  DataStoreName=SciRxPrevLoopDataUnread
  wires:
  Constant/1 -> Data Store Write/1
  Data Store Read3/1 -> Add/1
  Data Store Read1/1 -> Add/2
  Add/1 -> Data Store Write1/1

== system CM745A_Sci30CfgAndUse/Sci30CfgAndUse/Sci30CfgAndUsePer1/If Action Subsystem2/While Iterator Subsystem/If Action Subsystem/If Action Subsystem1 ==
  Action Port : ActionPort  ActionType=else
  Constant : Constant  OutDataTypeStr=uint8
  CopyRight2 : Subsystem  Description=|  mask(Copyright Information){none=on}
      | Copyright info block.                                               
      |                                                                     
      | Place copyright information at the top of every subsystem in design.
      mask prompts: none "No parameters"
      mask help: Place copyright information at the top of every subsystem in design.
      mask Display:
      | NxtrConf = 'Nexteer Confidential';
      | 
      | sys = bdroot; %handle for the current model ("system")
      | first = get_param(sys,'Created');
      | first = first(end-3:end);  %year is last four digits
      | 
      | last = get_param(sys,'LastModifiedDate');
      | if isempty(last)
      |     last = datestr(now,'yyyy');
      | else
      |     last = last(end-3:end);
      | end
      | 
      | if strcmp(first,last)
      |     fprintf('%s -- Copyright %s Nexteer',NxtrConf,first)
      | else
      |     fprintf('%s -- %s%s- %s Nexteer',NxtrConf,char(169),first,last)
      | end
  Data Store Read2 : DataStoreRead  DataStoreName=SciRxProcIdx
  Data Store Write : DataStoreWrite  DataStoreName=SciRxProcIdx
  RollovrAdd : Subsystem
  wires:
  Data Store Read2/1 -> RollovrAdd/1(In1)
  Constant/1 -> RollovrAdd/2(In2)
  RollovrAdd/1(Out1) -> Data Store Write/1

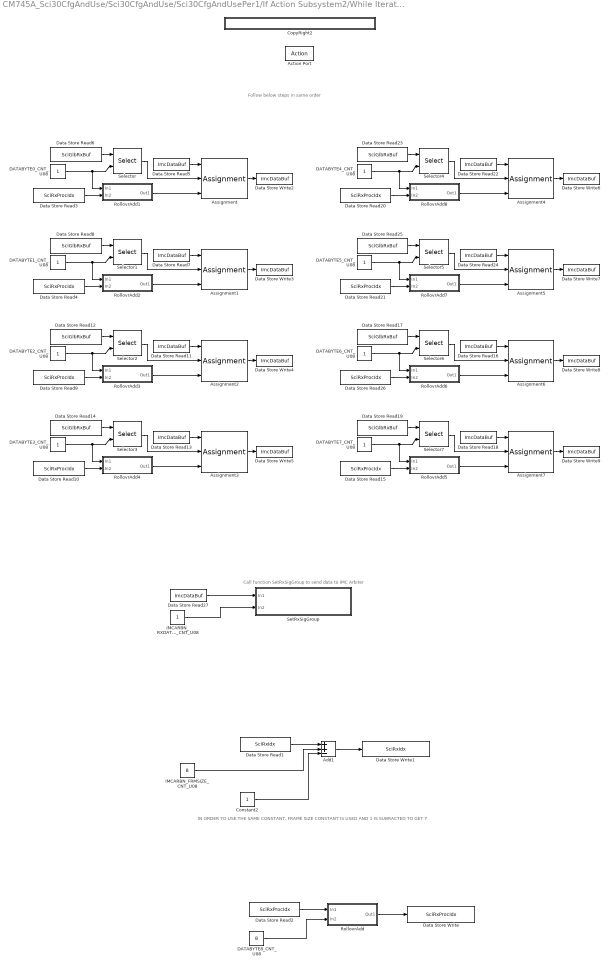
== system CM745A_Sci30CfgAndUse/Sci30CfgAndUse/Sci30CfgAndUsePer1/If Action Subsystem2/While Iterator Subsystem/If Action Subsystem/If Action Subsystem2 ==
  note: IN ORDER TO USE THE SAME CONSTANT, FRAME SIZE CONSTANT IS USED AND 1 IS SUBRACTED TO GET 7
  note: Call function SetRxSigGroup to send data to IMC Arbiter
  note: Follow below steps in same order
  Action Port : ActionPort  ActionType=elseif
  Add1 : Sum  Inputs=++-
  Assignment{,1..7} (8 alike) : Assignment  IndexMode=Zero-based  IndexOptions=Index vector (port)  Indices=1  OutputSizes=1
  Constant2 : Constant  OutDataTypeStr=uint8
  CopyRight2 : Subsystem  Description=|  mask(Copyright Information){none=on}
      | Copyright info block.                                               
      |                                                                     
      | Place copyright information at the top of every subsystem in design.
      mask prompts: none "No parameters"
      mask help: Place copyright information at the top of every subsystem in design.
      mask Display:
      | NxtrConf = 'Nexteer Confidential';
      | 
      | sys = bdroot; %handle for the current model ("system")
      | first = get_param(sys,'Created');
      | first = first(end-3:end);  %year is last four digits
      | 
      | last = get_param(sys,'LastModifiedDate');
      | if isempty(last)
      |     last = datestr(now,'yyyy');
      | else
      |     last = last(end-3:end);
      | end
      | 
      | if strcmp(first,last)
      |     fprintf('%s -- Copyright %s Nexteer',NxtrConf,first)
      | else
      |     fprintf('%s -- %s%s- %s Nexteer',NxtrConf,char(169),first,last)
      | end
  DATABYTE0_CNT_U08 : Constant
  DATABYTE1_CNT_U08 : Constant
  DATABYTE2_CNT_U08 : Constant
  DATABYTE3_CNT_U08 : Constant
  DATABYTE4_CNT_U08 : Constant
  DATABYTE5_CNT_U08 : Constant
  DATABYTE6_CNT_U08 : Constant
  DATABYTE7_CNT_U08 : Constant
  DATABYTE8_CNT_U08 : Constant  Value=8  OutDataTypeStr=uint8
  Data Store Read1 : DataStoreRead  DataStoreName=SciRxIdx
  Data Store Read{2..4,9..10,15,20..21,26} (9 alike) : DataStoreRead  DataStoreName=SciRxProcIdx
  Data Store Read{5,7,11,13,16,18,22,24,27} (9 alike) : DataStoreRead  DataStoreName=ImcDataBuf
  Data Store Read{6,8,12,14,17,19,23,25} (8 alike) : DataStoreRead  DataStoreName=SciGlbRxBuf
  Data Store Write : DataStoreWrite  DataStoreName=SciRxProcIdx
  Data Store Write1 : DataStoreWrite  DataStoreName=SciRxIdx
  Data Store Write{2..9} (8 alike) : DataStoreWrite  DataStoreName=ImcDataBuf
  IMCARBN_FRMSIZE_CNT_U08 : Constant  Value=8  OutDataTypeStr=uint8
  IMCARBN_RXDATASRC_CNT_U08 : Constant
  RollovrAdd : Subsystem
  RollovrAdd1 : Subsystem
  RollovrAdd2 : Subsystem
  RollovrAdd3 : Subsystem
  RollovrAdd4 : Subsystem
  RollovrAdd5 : Subsystem
  RollovrAdd6 : Subsystem
  RollovrAdd7 : Subsystem
  RollovrAdd8 : Subsystem
  Selector{,1..7} (8 alike) : Selector  IndexMode=Zero-based  InputPortWidth=8  IndexOptions=Index vector (port)  Indices=[1 3]  OutputSizes=1
  SetRxSigGroup : Subsystem
  wires:
  Data Store Read2/1 -> RollovrAdd/1(In1)
  IMCARBN_FRMSIZE_CNT_U08/1 -> Add1/2
  RollovrAdd/1(Out1) -> Data Store Write/1
  Data Store Read1/1 -> Add1/1
  Add1/1 -> Data Store Write1/1
  Constant2/1 -> Add1/3
  Assignment/1 -> Data Store Write2/1
  DATABYTE0_CNT_U08/1 -> RollovrAdd1/1(In1), Selector/2
  Data Store Read5/1 -> Assignment/1
  Selector/1 -> Assignment/2
  Data Store Read6/1 -> Selector/1
  RollovrAdd1/1(Out1) -> Assignment/3
  Data Store Read3/1 -> RollovrAdd1/2(In2)
  Assignment1/1 -> Data Store Write3/1
  DATABYTE1_CNT_U08/1 -> RollovrAdd2/1(In1), Selector1/2
  Data Store Read7/1 -> Assignment1/1
  Selector1/1 -> Assignment1/2
  Data Store Read8/1 -> Selector1/1
  RollovrAdd2/1(Out1) -> Assignment1/3
  Data Store Read4/1 -> RollovrAdd2/2(In2)
  Assignment2/1 -> Data Store Write4/1
  DATABYTE2_CNT_U08/1 -> RollovrAdd3/1(In1), Selector2/2
  Data Store Read11/1 -> Assignment2/1
  Selector2/1 -> Assignment2/2
  Data Store Read12/1 -> Selector2/1
  RollovrAdd3/1(Out1) -> Assignment2/3
  Data Store Read9/1 -> RollovrAdd3/2(In2)
  Assignment3/1 -> Data Store Write5/1
  DATABYTE3_CNT_U08/1 -> RollovrAdd4/1(In1), Selector3/2
  Data Store Read13/1 -> Assignment3/1
  Selector3/1 -> Assignment3/2
  Data Store Read14/1 -> Selector3/1
  RollovrAdd4/1(Out1) -> Assignment3/3
  Data Store Read10/1 -> RollovrAdd4/2(In2)
  Assignment4/1 -> Data Store Write6/1
  DATABYTE4_CNT_U08/1 -> RollovrAdd8/1(In1), Selector4/2
  Data Store Read22/1 -> Assignment4/1
  Selector4/1 -> Assignment4/2
  Data Store Read23/1 -> Selector4/1
  RollovrAdd8/1(Out1) -> Assignment4/3
  Data Store Read20/1 -> RollovrAdd8/2(In2)
  Assignment5/1 -> Data Store Write7/1
  DATABYTE5_CNT_U08/1 -> RollovrAdd7/1(In1), Selector5/2
  Data Store Read24/1 -> Assignment5/1
  Selector5/1 -> Assignment5/2
  Data Store Read25/1 -> Selector5/1
  RollovrAdd7/1(Out1) -> Assignment5/3
  Data Store Read21/1 -> RollovrAdd7/2(In2)
  Assignment6/1 -> Data Store Write8/1
  DATABYTE6_CNT_U08/1 -> RollovrAdd6/1(In1), Selector6/2
  Data Store Read16/1 -> Assignment6/1
  Selector6/1 -> Assignment6/2
  Data Store Read17/1 -> Selector6/1
  RollovrAdd6/1(Out1) -> Assignment6/3
  Data Store Read26/1 -> RollovrAdd6/2(In2)
  Assignment7/1 -> Data Store Write9/1
  DATABYTE7_CNT_U08/1 -> RollovrAdd5/1(In1), Selector7/2
  Data Store Read18/1 -> Assignment7/1
  Selector7/1 -> Assignment7/2
  Data Store Read19/1 -> Selector7/1
  RollovrAdd5/1(Out1) -> Assignment7/3
  Data Store Read15/1 -> RollovrAdd5/2(In2)
  Data Store Read27/1 -> SetRxSigGroup/1(In1)
  IMCARBN_RXDATASRC_CNT_U08/1 -> SetRxSigGroup/2(In2)
  DATABYTE8_CNT_U08/1 -> RollovrAdd/2(In2)

== system CM745A_Sci30CfgAndUse/Sci30CfgAndUse/Sci30CfgAndUsePer1/If Action Subsystem2/While Iterator Subsystem/If Action Subsystem/RollovrAdd ==
  In1 : Inport
  In2 : Inport  Port=2
  Add : Sum
  Constant : Constant  Value=2  OutDataTypeStr=uint8
  CopyRight2 : Subsystem  Description=|  mask(Copyright Information){none=on}
      | Copyright info block.                                               
      |                                                                     
      | Place copyright information at the top of every subsystem in design.
      mask prompts: none "No parameters"
      mask help: Place copyright information at the top of every subsystem in design.
      mask Display:
      | NxtrConf = 'Nexteer Confidential';
      | 
      | sys = bdroot; %handle for the current model ("system")
      | first = get_param(sys,'Created');
      | first = first(end-3:end);  %year is last four digits
      | 
      | last = get_param(sys,'LastModifiedDate');
      | if isempty(last)
      |     last = datestr(now,'yyyy');
      | else
      |     last = last(end-3:end);
      | end
      | 
      | if strcmp(first,last)
      |     fprintf('%s -- Copyright %s Nexteer',NxtrConf,first)
      | else
      |     fprintf('%s -- %s%s- %s Nexteer',NxtrConf,char(169),first,last)
      | end
  IMCARBN_FRMSIZE_CNT_U08 : Constant  Value=8
  MAXSIGGROUPFORTX_CNT_U08 : Constant  Value=9
  Math Function : Math  Operator=mod  SaturateOnIntegerOverflow=on
  Product : Product
  Product1 : Product
  Out1 : Outport
  wires:
  Math Function/1 -> Out1/1
  In1/1 -> Add/1
  In2/1 -> Add/2
  Add/1 -> Math Function/1
  Constant/1 -> Product/1
  IMCARBN_FRMSIZE_CNT_U08/1 -> Product/2
  Product/1 -> Product1/1
  Product1/1 -> Math Function/2
  MAXSIGGROUPFORTX_CNT_U08/1 -> Product1/2

== system CM745A_Sci30CfgAndUse/Sci30CfgAndUse/Sci30CfgAndUsePer1/If Action Subsystem2/While Iterator Subsystem/If Action Subsystem1/CopyRight2 ==

== system CM745A_Sci30CfgAndUse/Sci30CfgAndUse/Sci30CfgAndUsePer1/If Action Subsystem2/While Iterator Subsystem/If Action Subsystem1/RollovrAdd ==
  In1 : Inport
  In2 : Inport  Port=2
  Add : Sum
  Constant : Constant  Value=2  OutDataTypeStr=uint8
  CopyRight2 : Subsystem  Description=|  mask(Copyright Information){none=on}
      | Copyright info block.                                               
      |                                                                     
      | Place copyright information at the top of every subsystem in design.
      mask prompts: none "No parameters"
      mask help: Place copyright information at the top of every subsystem in design.
      mask Display:
      | NxtrConf = 'Nexteer Confidential';
      | 
      | sys = bdroot; %handle for the current model ("system")
      | first = get_param(sys,'Created');
      | first = first(end-3:end);  %year is last four digits
      | 
      | last = get_param(sys,'LastModifiedDate');
      | if isempty(last)
      |     last = datestr(now,'yyyy');
      | else
      |     last = last(end-3:end);
      | end
      | 
      | if strcmp(first,last)
      |     fprintf('%s -- Copyright %s Nexteer',NxtrConf,first)
      | else
      |     fprintf('%s -- %s%s- %s Nexteer',NxtrConf,char(169),first,last)
      | end
  IMCARBN_FRMSIZE_CNT_U08 : Constant  Value=8
  MAXSIGGROUPFORTX_CNT_U08 : Constant  Value=9
  Math Function : Math  Operator=mod  SaturateOnIntegerOverflow=on
  Product : Product  OutDataTypeStr=uint8
  Product1 : Product  OutDataTypeStr=uint8
  Out1 : Outport
  wires:
  Math Function/1 -> Out1/1
  In1/1 -> Add/1
  In2/1 -> Add/2
  Add/1 -> Math Function/1
  Constant/1 -> Product/1
  IMCARBN_FRMSIZE_CNT_U08/1 -> Product/2
  Product/1 -> Product1/1
  Product1/1 -> Math Function/2
  MAXSIGGROUPFORTX_CNT_U08/1 -> Product1/2

== system CM745A_Sci30CfgAndUse/Sci30CfgAndUse/Sci30CfgAndUsePer1/If Action Subsystem2/While Iterator Subsystem/RollovrAdd/CopyRight2 ==

== system CM745A_Sci30CfgAndUse/Sci30CfgAndUse/Sci30CfgAndUsePer2/Sci30Transmit/If Action Subsystem/While Iterator Subsystem/CopyRight2 ==

== system CM745A_Sci30CfgAndUse/Sci30CfgAndUse/Sci30CfgAndUsePer2/Sci30Transmit/If Action Subsystem1/If Action Subsystem/CopyRight2 ==
